simulink library "dynamics_lib"  (R2016b)
settings: Solver=ode45  StartTime=0.0  StopTime=10.0  RelTol=1e-3  EnableMultiTasking=on
undefined symbols (not defined in the file or in its folder): body_rates, position, quaternion, sim_params, velocity
libraries: aerolibutil x6, vrlib x1, bus_stubs_template x1
settings Model: Creator=bbarz_000  LastModifiedBy=taylorreynolds
settings DataIOCC: LimitDataPoints=on
settings OptimizationCC: LifeSpan=inf
settings DebuggingCC: AllowSymbolicDim=off  SFUnexpectedBacktrackingDiag=warning  SFNoUnconditionalDefaultTransitionDiag=warning  SFExecutionAtInitializationDiag=none
settings GRTTargetCC: TargetLangStandard=C89/C90 (ANSI)  GeneratePreprocessorConditionals=Disable all
settings ConfigComp: CovMetricSettings=dw  CovHtmlReporting=on  CovSaveCumulativeToWorkspaceVar=on  CovSaveSingleToWorkspaceVar=on  CovExternalEMLEnable=off

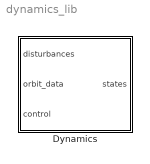
== system dynamics_lib ==
  Dynamics : Subsystem

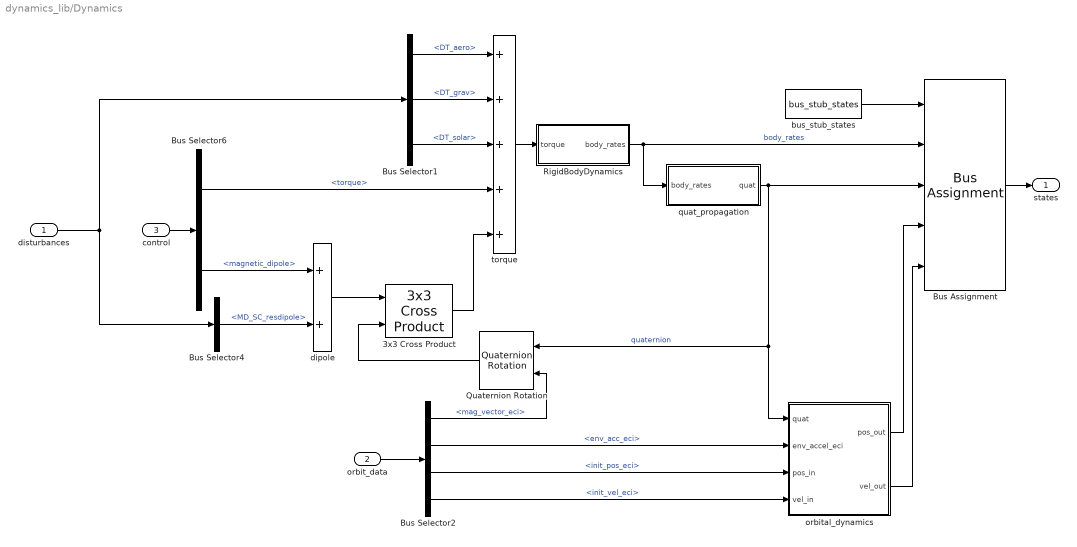
== system dynamics_lib/Dynamics ==
  disturbances : Inport  OutDataTypeStr=Bus: disturbances
  orbit_data : Inport  Port=2  OutDataTypeStr=Bus: orbit_data
  control : Inport  Port=3  OutDataTypeStr=Bus: control
  3x3 Cross Product : aerolibutil/3x3 Cross Product
  Bus Assignment : BusAssignment  AssignedSignals=body_rates,quaternion,position,velocity
  Bus Selector1 : BusSelector  OutputSignals=DT_aero,DT_grav,DT_solar
  Bus Selector2 : BusSelector  OutputSignals=mag_vector_eci,env_acc_eci,init_pos_eci,init_vel_eci
  Bus Selector4 : BusSelector  OutputSignals=MD_SC_resdipole
  Bus Selector6 : BusSelector  OutputSignals=torque,magnetic_dipole
  Quaternion Rotation : aerolibutil/Quaternion Rotation
  RigidBodyDynamics : Subsystem
  bus_stub_states : bus_stubs_template/bus_stub_states
  dipole : Sum  Inputs=2
  orbital_dynamics : Subsystem
  quat_propagation : Subsystem
  torque : Sum  Inputs=5
  states : Outport
  wires:
  Bus Assignment/1 -> states/1
  bus_stub_states/1 -> Bus Assignment/1
  quat_propagation/1(quat) -> Bus Assignment/3, orbital_dynamics/1(quat), Quaternion Rotation/1  "quaternion"
  RigidBodyDynamics/1(body_rates) -> Bus Assignment/2, quat_propagation/1(body_rates)  "body_rates"
  disturbances/1 -> Bus Selector4/1, Bus Selector1/1
  Bus Selector1/1 -> torque/1  "<DT_aero>"
  Bus Selector1/2 -> torque/2  "<DT_grav>"
  Bus Selector1/3 -> torque/3  "<DT_solar>"
  control/1 -> Bus Selector6/1
  Bus Selector6/1 -> torque/4  "<torque>"
  Bus Selector4/1 -> dipole/2  "<MD_SC_resdipole>"
  Bus Selector6/2 -> dipole/1  "<magnetic_dipole>"
  torque/1 -> RigidBodyDynamics/1(torque)
  dipole/1 -> 3x3 Cross Product/1
  Quaternion Rotation/1 -> 3x3 Cross Product/2
  3x3 Cross Product/1 -> torque/5
  Bus Selector2/2 -> orbital_dynamics/2(env_accel_eci)  "<env_acc_eci>"
  Bus Selector2/1 -> Quaternion Rotation/2  "<mag_vector_eci>"
  orbital_dynamics/2(vel_out) -> Bus Assignment/5
  orbital_dynamics/1(pos_out) -> Bus Assignment/4
  Bus Selector2/3 -> orbital_dynamics/3(pos_in)  "<init_pos_eci>"
  Bus Selector2/4 -> orbital_dynamics/4(vel_in)  "<init_vel_eci>"
  orbit_data/1 -> Bus Selector2/1

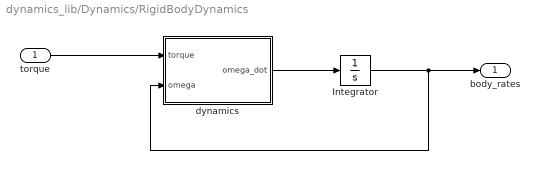
== system dynamics_lib/Dynamics/RigidBodyDynamics ==
  torque : Inport
  Integrator : Integrator  InitialCondition=sim_params.dynamics.ic.rate_init
  dynamics : Subsystem
  body_rates : Outport
  wires:
  dynamics/1(omega_dot) -> Integrator/1
  torque/1 -> dynamics/1(torque)
  Integrator/1 -> dynamics/2(omega), body_rates/1

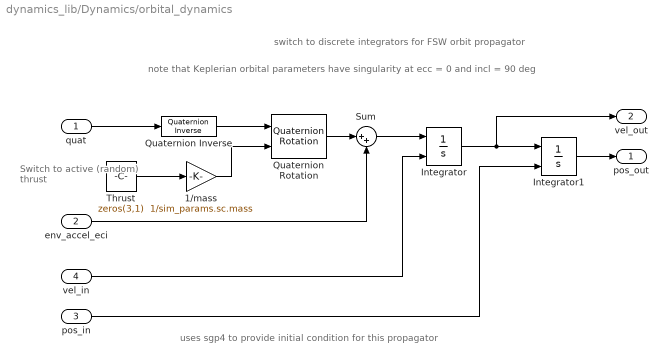
== system dynamics_lib/Dynamics/orbital_dynamics ==
  note: Switch to active
      | (random) thrust
  note: uses sgp4 to provide initial condition for this propagator
  note: note that Keplerian orbital parameters have singularity at ecc = 0 and incl = 90 deg
  note: switch to discrete integrators for FSW orbit propagator
  quat : Inport
  env_accel_eci : Inport  Port=2
  pos_in : Inport  Port=3
  vel_in : Inport  Port=4
  1/mass : Gain  Gain=1/sim_params.sc.mass
  Integrator : Integrator  InitialConditionSource=external  InitialCondition=sim_params.orbit.init_vel_eci
  Integrator1 : Integrator  InitialConditionSource=external  InitialCondition=sim_params.orbit.init_pos_eci
  Quaternion Inverse : aerolibutil/Quaternion Inverse
  Quaternion Rotation : aerolibutil/Quaternion Rotation
  Sum : Sum  Inputs=|++
  Thrust : Constant  Value=zeros(3,1)
  pos_out : Outport
  vel_out : Outport  Port=2
  wires:
  env_accel_eci/1 -> Sum/2
  Integrator/1 -> vel_out/1, Integrator1/1
  Thrust/1 -> 1/mass/1
  Sum/1 -> Integrator/1
  1/mass/1 -> Quaternion Rotation/2
  Quaternion Inverse/1 -> Quaternion Rotation/1
  Quaternion Rotation/1 -> Sum/1
  vel_in/1 -> Integrator/2
  pos_in/1 -> Integrator1/2
  quat/1 -> Quaternion Inverse/1
  Integrator1/1 -> pos_out/1

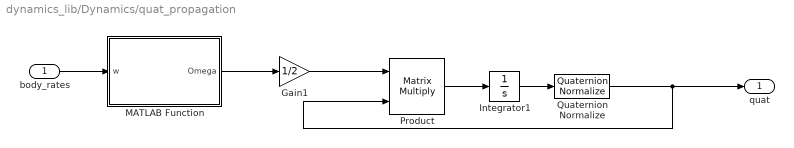
== system dynamics_lib/Dynamics/quat_propagation ==
  body_rates : Inport
  Gain1 : Gain  Gain=1/2
  Integrator1 : Integrator  InitialCondition=sim_params.dynamics.ic.quat_init
  MATLAB Function : MATLAB Function  TreatAsAtomicUnit=on
  Product : Product  Multiplication=Matrix(*)  RndMeth=Zero
  Quaternion Normalize : aerolibutil/Quaternion Normalize
  quat : Outport
  wires:
  MATLAB Function/1(Omega) -> Gain1/1
  body_rates/1 -> MATLAB Function/1(w)
  Quaternion Normalize/1 -> Product/2, quat/1
  Gain1/1 -> Product/1
  Integrator1/1 -> Quaternion Normalize/1
  Product/1 -> Integrator1/1

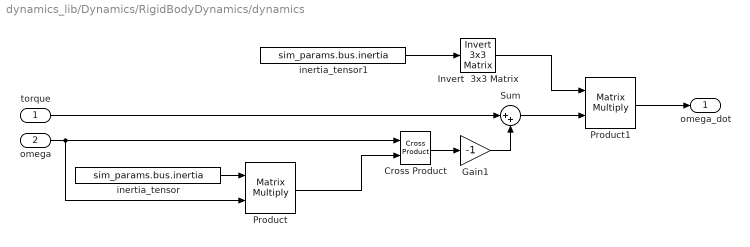
== system dynamics_lib/Dynamics/RigidBodyDynamics/dynamics ==
  torque : Inport
  omega : Inport  Port=2
  Cross Product : vrlib/Utilities/Cross Product
  Gain1 : Gain  Gain=-1
  Invert  3x3 Matrix : aerolibutil/Invert  3x3 Matrix
  Product : Product  Multiplication=Matrix(*)  RndMeth=Zero
  Product1 : Product  Multiplication=Matrix(*)  RndMeth=Zero
  Sum : Sum  Inputs=|++
  inertia_tensor : Constant  Value=sim_params.bus.inertia
  inertia_tensor1 : Constant  Value=sim_params.bus.inertia
  omega_dot : Outport
  wires:
  torque/1 -> Sum/1
  omega/1 -> Cross Product/1, Product/2
  inertia_tensor/1 -> Product/1
  Cross Product/1 -> Gain1/1
  Product/1 -> Cross Product/2
  Sum/1 -> Product1/2
  Product1/1 -> omega_dot/1
  Invert  3x3 Matrix/1 -> Product1/1
  inertia_tensor1/1 -> Invert  3x3 Matrix/1
  Gain1/1 -> Sum/2

== matlab function dynamics_lib/Dynamics/quat_propagation/MATLAB Function ==
  data: w input; Omega output
function Omega = skew_sym(w)
%#codegen

    w_skew = ...
        [0 w(3) -w(2);
        -w(3) 0 w(1);
        w(2) -w(1) 0];

    Omega = ...
        [0 -w';
        w w_skew];
